simulink model "Simulacion_stepper_2024a"  (R2024a)
settings: Solver=ode4  StartTime=0.0  StopTime=Time_simulation  FixedStep=1/frecuency_simulation  RelTol=1e-3
InitFcn:
  | %%InitFcn();
StopFcn:
  | %%FinishFcn
model workspace (MAT data in the model file):
  Ts_stepper = 0.001
values from neighbouring files (symbols this model uses):
  B = motor_params.B_internal    [bode.m]    (also in current_observer.m = 0.0005; discretizacion.m = [ 1/L, 0; ekf_4_estados.m = params.B; obs_ctrl_back_emf_ext.m = [1/L 0)
  B0 = 3*wn_w - BJ_hat    [Barrido_B.m]    (also in Barrido_J.m; InitFcn.m = 449.962302294)
  B1 = 3*wn_w^2 - B0*BJ_hat    [Barrido_B.m]    (also in Barrido_J.m; InitFcn.m = 64448.3670019)
  B2 = -(J_var/P)*(wn_w^3)    [Barrido_B.m]    (also in Barrido_J.m; InitFcn.m = -0.364323750994)
  B_internal = 1e-4    (= 0.0001)    [InitFcn.m]
  B_var = B_internal* B_factors(k)    [Barrido_B.m]    (also in Barrido_J.m = B_real; InitFcn.m = 0.0001)
  frecuency_simulation = 10e3    (= 10000)    [InitFcn.m]
  I_nom = 1    [InitFcn.m]    (also in salient_motor.m)
  J = motor_params.J_internal    [bode.m]    (also in current_observer.m = 0.008; ekf_4_estados.m = params.J; obs_ctrl_back_emf_ext.m = 0.008; obs_y_contrl_back_emd.m = 0.008)
  J_internal = 4.7/1000000    (= 4.7e-06)    [InitFcn.m]
  J_var = J_real    [Barrido_B.m]    (also in Barrido_J.m = J_internal * J_factors(k); InitFcn.m = 4.7e-06)
  Ke = Kt    [InitFcn.m]    (also in current_observer.m = 0.0055; ekf_4_estados.m = params.Ke; observer.m = Pvec(3); salient_motor.m = 0.0066)
  Ki_d = wd_d*R    (= 3926.99081699)    [InitFcn.m]    (also in bode.m = PI_dq_params.Ki_d_salient)
  Ki_d_salient = wd_d^2*Ld    (= 21491.0635834)    [InitFcn.m]
  Ki_q = wd_q*R    (= 3926.99081699)    [InitFcn.m]    (also in bode.m = PI_dq_params.Ki_q_salient)
  Ki_q_salient = wd_q^2*Lq    (= 7846.33549887)    [InitFcn.m]
  Ki_w = (wn_w^2)*J_var/Kt    [Barrido_B.m]    (also in Barrido_J.m; InitFcn.m; bode.m = PI_MTPA_params.Ki_w)
  Kp_d = wd_d*L    (= 9.42477796077)    [InitFcn.m]    (also in bode.m = PI_dq_params.Kp_d_salient)
  Kp_d_salient = 2*shi_d*wd_d*Ld -R    (= 16.845833313)    [InitFcn.m]
  Kp_q = wd_q*L    (= 9.42477796077)    [InitFcn.m]    (also in bode.m = PI_dq_params.Kp_q_salient)
  Kp_q_salient = 2*shi_q*wd_q*Lq-R    (= 4.56311709936)    [InitFcn.m]
  Kp_w = (2*shi_w*wn_w*J_var)/Kt    [Barrido_B.m]    (also in Barrido_J.m; InitFcn.m; bode.m = PI_MTPA_params.Kp_w)
  Kt = Thold / (sqrt(2) * I_nom)    [InitFcn.m]    (also in current_observer.m = 0.275; ekf_4_estados.m = params.Kt; frecuencia_max.m = 0.33; observer.m = Pvec(4))
  L = 6/1000    (= 0.006)    [InitFcn.m]    (also in current_observer.m = place(A', C', 10*eig(A)).'; desfase.m = lags(k); discretizacion.m = 0.01; frecuencia_max.m)
  Ld = L0 + L2    [Copy_of_PMSM_salient.m]    (also in InitFcn.m = 0.00871; bode.m = motor_params.Ld; ekf_4_estados.m = params.Ld; salient_motor.m = 0.00871)
  Lq = L0 - L2    [Copy_of_PMSM_salient.m]    (also in InitFcn.m = 0.00318; bode.m = motor_params.Lq; ekf_4_estados.m = params.Lq; salient_motor.m = 0.00318)
  N_steps = 360/Step_angle    (= 200)    [InitFcn.m]
  P = N_teeths/2    (= 50)    [InitFcn.m]    (also in bode.m = motor_params.P; ekf_4_estados.m = P_pred; frecuencia_max.m; salient_motor.m)
  Phi = pi/2    (= 1.57079632679)    [InitFcn.m]    (also in ekf_4_estados.m = eye(4) + Ts_eff*A)
  Psi = Kt/P    [InitFcn.m]    (also in bode.m = motor_params.Ke; salient_motor.m = 0.0066)
  R = 2.5    [InitFcn.m]    (also in bode.m = motor_params.R; current_observer.m = 3.4; discretizacion.m = 3.4; ekf_4_estados.m = params.R)
  sample_time = 1/frecuency_simulation    (= 0.0001)    [InitFcn.m]
  Tdm = 18/1000    (= 0.018)    [InitFcn.m]    (also in salient_motor.m)
  Ts_current = 1/f_current    (= 0.0001)    [InitFcn.m]
  Ts_DO = Ts_Wm    (= 0.0001)    [InitFcn.m]
  Ts_ekf = 1/f_ekf    (= 0.0001)    [InitFcn.m]
  Ts_Wm = Ts_current    (= 0.0001)    [InitFcn.m]
  Vdc = 12    [InitFcn.m]    (also in frecuencia_max.m)
undefined symbols (not defined in the file or in its folder): DiscIntNeverNeededParam
libraries: fl_lib x27, nesl_utility x19, spsMosfetLib x16, simulink x8, eeTransforms x4, spsDCVoltageSourceLib x4, spsVoltageMeasurementLib x4, ee_lib x3, slexportprevious_tp74def212_4eb8_4616_a2bc_f4e795655e99 x1, spsTriangleGeneratorLib x1, spspowerguiLib x1
(part 2 of 4)

== system Simulacion_stepper_2024a/Meas 1 ==
  ERef : fl_lib/Electrical/Electrical Elements/Electrical Reference
  PS-Simulink Converter : nesl_utility/PS-Simulink Converter  PhysicalDomain=network_engine_domain  SubClassName=ps_output  LeftPortType=input  RightPortType=output  PseudoPeriodic=off  Frequencies=[]  VectorFormat=1-D array  Unit=V  AffineConversion=off
  Voltage Sensor : fl_lib/Electrical/Electrical Sensors/Voltage Sensor
  V : PMIOPort  Side=Left
  SL : Outport  VectorParamsAs1DForOutWhenUnconnected=off
  wires:
  PS-Simulink Converter/1 -> SL/1
  connections:
  V/RConn1 -- Voltage Sensor/LConn1
  ERef/LConn1 -- Voltage Sensor/RConn2
  Voltage Sensor/RConn1 -- PS-Simulink Converter/LConn1

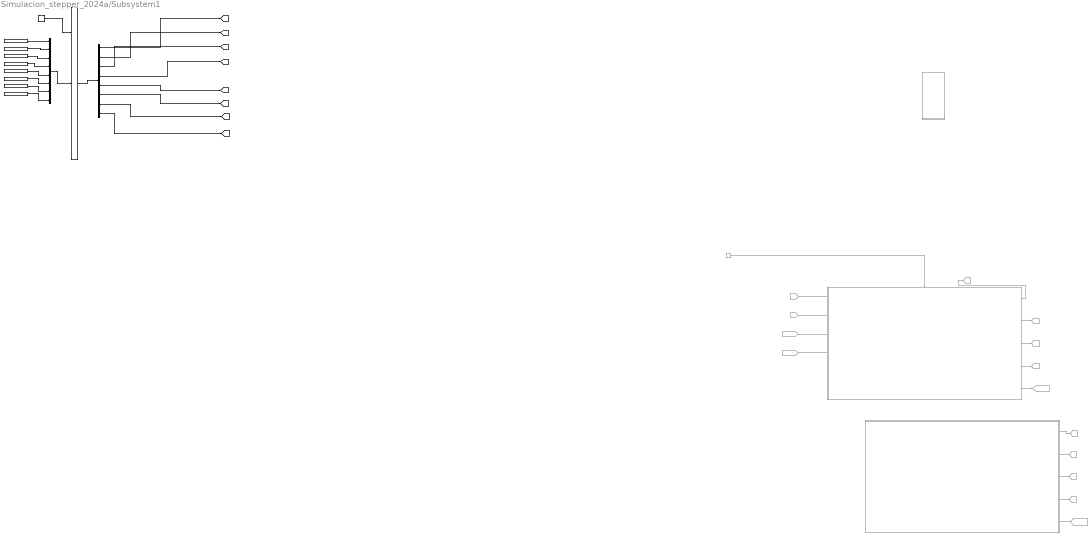
== system Simulacion_stepper_2024a/Subsystem1 ==
  note: A
  note: A
  note: A
  Constant1 : Constant
  Demux6 : Demux  Outputs=8
  From103 : From  Commented=on  GotoTag=Ib_M1
  From110 : From  Commented=on  GotoTag=Wm_ref  TagVisibility=global
  From112 : From  Commented=on  GotoTag=Wm_planta_M1  TagVisibility=global
  From98 : From  Commented=on  GotoTag=Ia_M1
  Function-Call Generator3 : FunctionCallGenerator  Commented=on  SampleTime=sample_time
  Goto14 : Goto  Commented=on  GotoTag=Vd_M2  TagVisibility=global
  Goto15 : Goto  Commented=on  GotoTag=Vq_M2  TagVisibility=global
  Goto16 : Goto  Commented=on  GotoTag=Iq_M2  TagVisibility=global
  Goto17 : Goto  Commented=on  GotoTag=Iq_ref_M2  TagVisibility=global
  Goto4 : Goto  Commented=on  GotoTag=Id_M2  TagVisibility=global
  Goto55 : Goto  Commented=on  GotoTag=Id_M1  TagVisibility=global
  Goto64 : Goto  Commented=on  GotoTag=Vd_M1  TagVisibility=global
  Goto65 : Goto  Commented=on  GotoTag=Vq_M1  TagVisibility=global
  Goto66 : Goto  Commented=on  GotoTag=Iq_M1  TagVisibility=global
  Goto68 : Goto  Commented=on  GotoTag=Iq_ref_M1  TagVisibility=global
  Multiport Switch : MultiPortSwitch  Inputs=2  SaturateOnIntegerOverflow=off  InputSameDT=off
  Mux1 : Mux  Inputs=8
  Repeating Sequence Stair : simulink/Sources/Repeating Sequence Stair  OutValues=[1 0 0 0]  tsamp=Ts_stepper  OutMin=[]  OutMax=[]  OutDataTypeStr=double  OutputDataTypeScalingMode=double  OutDataType=fixdt(0,8)  ConRadixGroup=Best Precision: Vector-wise  OutScaling=2^-12
  Repeating Sequence Stair1 : simulink/Sources/Repeating Sequence Stair  OutValues=[1 0 1 0]  tsamp=Ts_stepper  OutMin=[]  OutMax=[]  OutDataTypeStr=double  OutputDataTypeScalingMode=double  OutDataType=fixdt(0,8)  ConRadixGroup=Best Precision: Vector-wise  OutScaling=2^-12
  Repeating Sequence Stair10 : simulink/Sources/Repeating Sequence Stair  OutValues=[0 0 0 1]  tsamp=Ts_stepper  OutMin=[]  OutMax=[]  OutDataTypeStr=double  OutputDataTypeScalingMode=double  OutDataType=fixdt(0,8)  ConRadixGroup=Best Precision: Vector-wise  OutScaling=2^-12
  Repeating Sequence Stair11 : simulink/Sources/Repeating Sequence Stair  OutValues=[1 0 0 1]  tsamp=Ts_stepper  OutMin=[]  OutMax=[]  OutDataTypeStr=double  OutputDataTypeScalingMode=double  OutDataType=fixdt(0,8)  ConRadixGroup=Best Precision: Vector-wise  OutScaling=2^-12
  Repeating Sequence Stair2 : simulink/Sources/Repeating Sequence Stair  OutValues=[0 0 1 0]  tsamp=Ts_stepper  OutMin=[]  OutMax=[]  OutDataTypeStr=double  OutputDataTypeScalingMode=double  OutDataType=fixdt(0,8)  ConRadixGroup=Best Precision: Vector-wise  OutScaling=2^-12
  Repeating Sequence Stair3 : simulink/Sources/Repeating Sequence Stair  OutValues=[0 1 1 0]  tsamp=Ts_stepper  OutMin=[]  OutMax=[]  OutDataTypeStr=double  OutputDataTypeScalingMode=double  OutDataType=fixdt(0,8)  ConRadixGroup=Best Precision: Vector-wise  OutScaling=2^-12
  Repeating Sequence Stair8 : simulink/Sources/Repeating Sequence Stair  OutValues=[0 1 0 0]  tsamp=Ts_stepper  OutMin=[]  OutMax=[]  OutDataTypeStr=double  OutputDataTypeScalingMode=double  OutDataType=fixdt(0,8)  ConRadixGroup=Best Precision: Vector-wise  OutScaling=2^-12
  Repeating Sequence Stair9 : simulink/Sources/Repeating Sequence Stair  OutValues=[0 1 0 1]  tsamp=Ts_stepper  OutMin=[]  OutMax=[]  OutDataTypeStr=double  OutputDataTypeScalingMode=double  OutDataType=fixdt(0,8)  ConRadixGroup=Best Precision: Vector-wise  OutScaling=2^-12
  Subsystem : Subsystem  Commented=on
  Triggered Subsystem2 : Subsystem  Commented=on  TreatAsAtomicUnit=on
  Triggered Subsystem4 : Subsystem  Commented=on  TreatAsAtomicUnit=on
  wires:
  Triggered Subsystem2/4(Iq) -> Goto66/1
  Triggered Subsystem2/1(Vd) -> Goto64/1
  ? -> Triggered Subsystem4/6(Tl_Tdm)
  ? -> Triggered Subsystem2/5(Theta)
  ? -> Triggered Subsystem4/3(Wm_ref)
  Triggered Subsystem2/5(Iq_ref) -> Goto68/1
  From112/1 -> Triggered Subsystem2/4(Wm)
  Triggered Subsystem4/2(Vq) -> Goto15/1
  From98/1 -> Triggered Subsystem2/1(Ia)
  Triggered Subsystem2/2(Vq) -> Goto65/1
  ? -> Triggered Subsystem2/6(Tl_Tdm)
  From103/1 -> Triggered Subsystem2/2(Ib)
  Triggered Subsystem2/3(Id) -> Goto55/1
  From110/1 -> Triggered Subsystem2/3(Wm_ref)
  Triggered Subsystem4/3(Id) -> Goto4/1
  ? -> Triggered Subsystem4/Trigger
  Triggered Subsystem4/4(Iq) -> Goto16/1
  ? -> Triggered Subsystem4/4(Wm)
  Triggered Subsystem4/5(Iq_ref) -> Goto17/1
  ? -> Triggered Subsystem4/5(Theta)
  ? -> Triggered Subsystem4/1(Ia)
  Function-Call Generator3/1 -> Triggered Subsystem2/Trigger
  ? -> Triggered Subsystem4/2(Ib)
  Triggered Subsystem4/1(Vd) -> Goto14/1
  Demux6/2 -> [S2_M0]
  Demux6/1 -> [S1_M0]
  Repeating Sequence Stair10/1 -> Mux1/7
  Repeating Sequence Stair8/1 -> Mux1/5
  Repeating Sequence Stair9/1 -> Mux1/6
  Demux6/8 -> [S8_M0]
  Demux6/4 -> [S4_M0]
  Demux6/7 -> [S7_M0]
  Demux6/6 -> [S6_M0]
  Constant1/1 -> Multiport Switch/1
  Repeating Sequence Stair/1 -> Mux1/1
  Mux1/1 -> Multiport Switch/2
  Repeating Sequence Stair3/1 -> Mux1/4
  Repeating Sequence Stair11/1 -> Mux1/8
  Demux6/5 -> [S5_M0]
  Repeating Sequence Stair2/1 -> Mux1/3
  Repeating Sequence Stair1/1 -> Mux1/2
  Multiport Switch/1 -> Demux6/1
  Demux6/3 -> [S3_M0]

== system Simulacion_stepper_2024a/Triggered Subsystem ==
  Wm_cmd : Inport
  Trigger : TriggerPort  TriggerType=function-call  VariantControl=(inherit)
  Constant : Constant  Value=1/1000
  Constant1 : Constant  Value=0
  MATLAB Function : MATLAB Function  TreatAsAtomicUnit=on
  Wm_ref : Outport
  Alpha_ref : Outport  Port=2
  wires:
  MATLAB Function/1(Wm_ref) -> Wm_ref/1
  MATLAB Function/2(alpha_ref) -> Alpha_ref/1
  Wm_cmd/1 -> MATLAB Function/1(Wm_cmd)
  Constant/1 -> MATLAB Function/2(Ts)
  Constant1/1 -> MATLAB Function/3(slope)

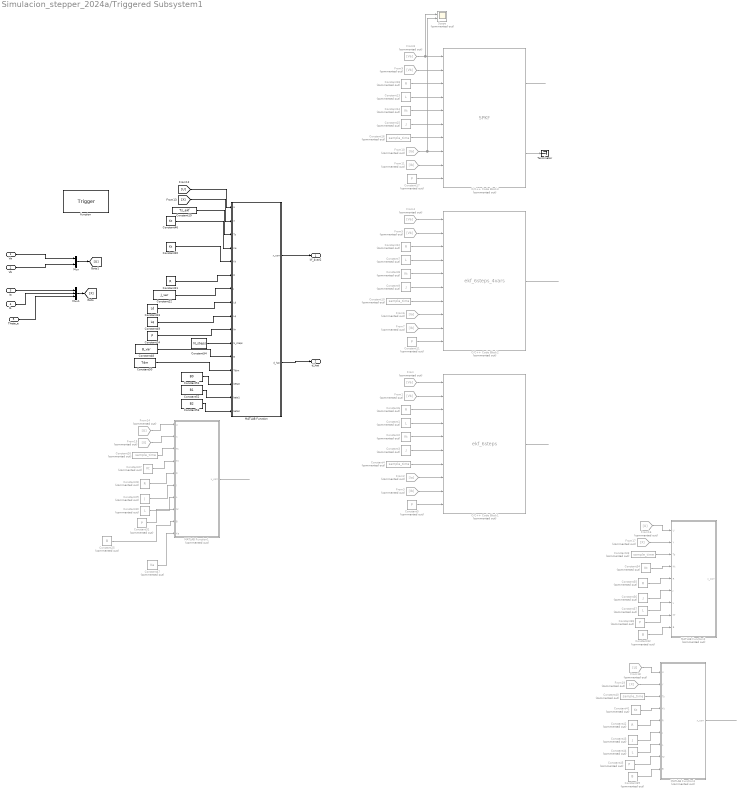
== system Simulacion_stepper_2024a/Triggered Subsystem1 ==
  Va : Inport
  Vb : Inport  Port=2
  Ia : Inport  Port=3
  Ib : Inport  Port=4
  Theta_e : Inport  Port=5
  function : TriggerPort  TriggerType=function-call  VariantControl=(inherit)  SampleTime=1/100
  C/C++ Code Block1 : S-Function  Commented=on  FunctionName=ekf_6steps  SFunctionModules=ekf_6steps_wrapper.c  SFunctionDeploymentMode=off  EnableBusSupport=off  mask(S-Function Builder){}
      mask help: Simulink:masks:SFunctionBuilder_MD
      mask init:
      | val = [[.9  0.75 0.75 1 1 .9 .9 1]',[1 1 0.75 0.75 .9 .9 1 .9]'];try , sys = get_param(gcb,'SfunBuilderFcnName');if isempty(sys), sys = get_param(gcb,'FunctionName'); end,catch, sys = get_param(gcb,'FunctionName'); end
      settings: CopyFcn=set_param(gcbh,'LinkStatus','none')  OpenFcn=sfunctionwizard(gcbh)
      mask Display:
      | plot(val(:,1),val(:,2))
      | disp(sys)
      | port_label('input',1,sprintf('%s', 'Va'),'interpreter','tex')
      | port_label('input',2,sprintf('%s', 'Vb'),'interpreter','tex')
      | port_label('input',3,sprintf('%s', 'R'),'interpreter','tex')
      | port_label('input',4,sprintf('%s', 'L'),'interpreter','tex')
      | port_label('input',5,sprintf('%s', 'Kt'),'interpreter','tex')
      | port_label('input',6,sprintf('%s', 'J'),'interpreter','tex')
      | port_label('input',7,sprintf('%s', 'Ts'),'interpreter','tex')
      | port_label('input',8,sprintf('%s', 'Ia\_medido'),'interpreter','tex')
      | port_label('input',9,sprintf('%s', 'Ib\_medido'),'interpreter','tex')
      | port_label('input',10,sprintf('%s', 'Nr'),'interpreter','tex')
      | port_label('output',1,sprintf('%s', 'x\_corr\_out'),'interpreter','tex')
  C/C++ Code Block2 : S-Function  Commented=on  FunctionName=ekf_6steps_4vars  SFunctionModules=ekf_6steps_4vars_wrapper.c  SFunctionDeploymentMode=off  EnableBusSupport=off  mask(S-Function Builder){}
      mask help: Simulink:masks:SFunctionBuilder_MD
      mask init: same as Simulacion_stepper_2024a/Triggered Subsystem1/C/C++ Code Block1
      settings: CopyFcn=set_param(gcbh,'LinkStatus','none')  OpenFcn=sfunctionwizard(gcbh)
      mask Display:
      | plot(val(:,1),val(:,2))
      | disp(sys)
      | port_label('input',1,sprintf('%s', 'Va'),'interpreter','tex')
      | port_label('input',2,sprintf('%s', 'Vb'),'interpreter','tex')
      | port_label('input',3,sprintf('%s', 'R'),'interpreter','tex')
      | port_label('input',4,sprintf('%s', 'L'),'interpreter','tex')
      | port_label('input',5,sprintf('%s', 'Kt'),'interpreter','tex')
      | port_label('input',6,sprintf('%s', 'J'),'interpreter','tex')
      | port_label('input',7,sprintf('%s', 'Ts'),'interpreter','tex')
      | port_label('input',8,sprintf('%s', 'Ia\_medido'),'interpreter','tex')
      | port_label('input',9,sprintf('%s', 'Ib\_medido'),'interpreter','tex')
      | port_label('input',10,sprintf('%s', 'Nr'),'interpreter','tex')
      | port_label('output',1,sprintf('%s', 'x\_corr\_out'),'interpreter','tex')
  C/C++ Code Block3 : S-Function  Commented=on  FunctionName=SPKF  SFunctionModules=SPKF_wrapper.c  SFunctionDeploymentMode=off  EnableBusSupport=off  mask(S-Function Builder){}
      mask help: Simulink:masks:SFunctionBuilder_MD
      mask init: same as Simulacion_stepper_2024a/Triggered Subsystem1/C/C++ Code Block1
      settings: CopyFcn=set_param(gcbh,'LinkStatus','none')  OpenFcn=sfunctionwizard(gcbh)
      mask Display:
      | plot(val(:,1),val(:,2))
      | disp(sys)
      | port_label('input',1,sprintf('%s', 'Va'),'interpreter','tex')
      | port_label('input',2,sprintf('%s', 'Vb'),'interpreter','tex')
      | port_label('input',3,sprintf('%s', 'R'),'interpreter','tex')
      | port_label('input',4,sprintf('%s', 'L'),'interpreter','tex')
      | port_label('input',5,sprintf('%s', 'Kt'),'interpreter','tex')
      | port_label('input',6,sprintf('%s', 'J'),'interpreter','tex')
      | port_label('input',7,sprintf('%s', 'Ts'),'interpreter','tex')
      | port_label('input',8,sprintf('%s', 'Ia\_medido'),'interpreter','tex')
      | port_label('input',9,sprintf('%s', 'Ib\_medido'),'interpreter','tex')
      | port_label('input',10,sprintf('%s', 'Nr'),'interpreter','tex')
      | port_label('output',1,sprintf('%s', 'x'),'interpreter','tex')
      | port_label('output',2,sprintf('%s', 'x\_aux'),'interpreter','tex')
  Constant{1,7,13,30,37,44} (6 alike) : Constant  Commented=on  Value=L  OutDataTypeStr=double
  Constant{4,10,16,26,33,40} (6 alike) : Constant  Commented=on  Value=sample_time  OutDataTypeStr=double
  Constant{5,11,17,31,38,45} (6 alike) : Constant  Commented=on  Value=P  OutDataTypeStr=double
  Constant{6,12,18,28,35,42} (6 alike) : Constant  Commented=on  Value=R  OutDataTypeStr=double
  Constant{2,8,14,27,34,41} (6 alike) : Constant  Commented=on  Value=Kt  OutDataTypeStr=double
  Constant{3,9,15,29,36,43} (6 alike) : Constant  Commented=on  Value=J  OutDataTypeStr=double
  Constant19 : Constant  Value=Ts_ekf  OutDataTypeStr=double
  Constant20 : Constant  Value=Kt  OutDataTypeStr=double
  Constant21 : Constant  Value=R  OutDataTypeStr=double
  Constant22 : Constant  Value=J_var  OutDataTypeStr=double
  Constant23 : Constant  Value=Ld  OutDataTypeStr=double
  Constant24 : Constant  Value=P  OutDataTypeStr=double
  Constant25 : Constant  Commented=on  Value=B
  Constant32 : Constant  Commented=on  Value=B
  Constant39 : Constant  Commented=on  Value=B
  Constant46 : Constant  Value=Kt  OutDataTypeStr=double
  Constant47 : Constant  Commented=on  Value=Ke  OutDataTypeStr=double
  Constant48 : Constant  Value=B_var  OutDataTypeStr=double
  Constant49 : Constant  Value=Lq  OutDataTypeStr=double
  Constant50 : Constant  Value=Tdm  OutDataTypeStr=double
  Constant51 : Constant  Value=B0  OutDataTypeStr=double
  Constant52 : Constant  Value=B1  OutDataTypeStr=double
  Constant53 : Constant  Value=B2  OutDataTypeStr=double
  Constant54 : Constant  Value=N_steps  OutDataTypeStr=double
  From : From  Commented=on  GotoTag=Va
  From1 : From  Commented=on  GotoTag=Vb
  From10 : From  Commented=on  GotoTag=Ia
  From11 : From  Commented=on  GotoTag=Ib
  From14 : From  Commented=on  GotoTag=U
  From15 : From  Commented=on  GotoTag=X
  From16 : From  Commented=on  GotoTag=U
  From17 : From  Commented=on  GotoTag=X
  From18 : From  Commented=on  GotoTag=U
  From19 : From  Commented=on  GotoTag=X
  From2 : From  Commented=on  GotoTag=Ia
  From3 : From  Commented=on  GotoTag=Ib
  From4 : From  Commented=on  GotoTag=Va
  From5 : From  Commented=on  GotoTag=Vb
  From6 : From  Commented=on  GotoTag=Ia
  From7 : From  Commented=on  GotoTag=Ib
  From8 : From  Commented=on  GotoTag=Va
  From9 : From  Commented=on  GotoTag=Vb
  MATLAB Function : MATLAB Function  TreatAsAtomicUnit=on
  MATLAB Function1 : MATLAB Function  Commented=on  TreatAsAtomicUnit=on
  MATLAB Function2 : MATLAB Function  Commented=on  TreatAsAtomicUnit=on
  MATLAB Function3 : MATLAB Function  Commented=on  TreatAsAtomicUnit=on
  Mux : Mux  Inputs=2
  Mux1 : Mux  Inputs=3
  Scope : Scope  Commented=on  NumInputPorts=2
  Terminator : Terminator
  kf_4var2 : Outport  PortDimensions=[4 1]
  d_hat : Outport  Port=2
  wires:
  Constant4/1 -> C/C++ Code Block1/7
  Constant5/1 -> C/C++ Code Block1/10
  C/C++ Code Block1/1 -> ?
  Constant6/1 -> C/C++ Code Block1/3
  Constant1/1 -> C/C++ Code Block1/4
  Constant2/1 -> C/C++ Code Block1/5
  Constant3/1 -> C/C++ Code Block1/6
  C/C++ Code Block2/1 -> ?
  C/C++ Code Block3/1 -> ?
  Vb/1 -> Mux/2
  Va/1 -> Mux/1
  Ib/1 -> Mux1/2
  Ia/1 -> Mux1/1
  From/1 -> C/C++ Code Block1/1
  From1/1 -> C/C++ Code Block1/2
  From2/1 -> C/C++ Code Block1/8
  From3/1 -> C/C++ Code Block1/9
  From4/1 -> C/C++ Code Block2/1
  From7/1 -> C/C++ Code Block2/9
  Constant8/1 -> C/C++ Code Block2/5
  Constant12/1 -> C/C++ Code Block2/3
  From5/1 -> C/C++ Code Block2/2
  Constant11/1 -> C/C++ Code Block2/10
  From6/1 -> C/C++ Code Block2/8
  Constant9/1 -> C/C++ Code Block2/6
  Constant7/1 -> C/C++ Code Block2/4
  Constant10/1 -> C/C++ Code Block2/7
  From8/1 -> Scope/1, C/C++ Code Block3/1
  From11/1 -> C/C++ Code Block3/9
  Constant14/1 -> C/C++ Code Block3/5
  Constant18/1 -> C/C++ Code Block3/3
  From9/1 -> C/C++ Code Block3/2
  Constant17/1 -> C/C++ Code Block3/10
  From10/1 -> Scope/2, C/C++ Code Block3/8
  Constant15/1 -> C/C++ Code Block3/6
  Constant13/1 -> C/C++ Code Block3/4
  Constant16/1 -> C/C++ Code Block3/7
  C/C++ Code Block3/2 -> Terminator/1
  Mux1/1 -> [X]
  Mux/1 -> [U]
  From16/1 -> MATLAB Function2/1(U)
  From17/1 -> MATLAB Function2/2(Y)
  Constant33/1 -> MATLAB Function2/3(Ts)
  Constant32/1 -> MATLAB Function2/9(B)
  Constant37/1 -> MATLAB Function2/7(L)
  Constant35/1 -> MATLAB Function2/5(R)
  Constant36/1 -> MATLAB Function2/6(J)
  Constant34/1 -> MATLAB Function2/4(Kt)
  Constant38/1 -> MATLAB Function2/8(Nr)
  MATLAB Function3/1(x_corr) -> ?
  Constant45/1 -> MATLAB Function3/8(Nr)
  Constant41/1 -> MATLAB Function3/4(Kt)
  From19/1 -> MATLAB Function3/2(Y)
  Constant43/1 -> MATLAB Function3/6(J)
  Constant40/1 -> MATLAB Function3/3(Ts)
  Constant39/1 -> MATLAB Function3/9(B)
  Constant42/1 -> MATLAB Function3/5(R)
  From18/1 -> MATLAB Function3/1(U)
  Constant44/1 -> MATLAB Function3/7(L)
  From15/1 -> MATLAB Function1/2(X)
  Constant27/1 -> MATLAB Function1/4(Kt)
  Constant31/1 -> MATLAB Function1/8(Nr)
  Constant29/1 -> MATLAB Function1/6(J)
  Constant25/1 -> MATLAB Function1/9(B)
  Constant26/1 -> MATLAB Function1/3(Ts)
  Constant30/1 -> MATLAB Function1/7(L)
  Constant28/1 -> MATLAB Function1/5(R)
  From14/1 -> MATLAB Function1/1(U)
  Constant47/1 -> MATLAB Function1/10(Ke)
  MATLAB Function1/1(x_corr) -> ?
  [U] -> MATLAB Function/1(U)
  [X] -> MATLAB Function/2(X)
  Constant19/1 -> MATLAB Function/3(Ts)
  Constant46/1 -> MATLAB Function/4(Ke)
  Constant20/1 -> MATLAB Function/5(Kt)
  Constant21/1 -> MATLAB Function/6(R)
  Constant22/1 -> MATLAB Function/7(J)
  Constant23/1 -> MATLAB Function/8(Ld)
  Constant49/1 -> MATLAB Function/9(Lq)
  Constant24/1 -> MATLAB Function/10(Nr)
  Constant48/1 -> MATLAB Function/12(B)
  Constant50/1 -> MATLAB Function/13(Tdtm)
  MATLAB Function/1(x_corr) -> kf_4var2/1
  Theta_e/1 -> Mux1/3
  Constant51/1 -> MATLAB Function/14(beta0)
  Constant52/1 -> MATLAB Function/15(beta1)
  Constant53/1 -> MATLAB Function/16(beta2)
  MATLAB Function/2(d_hat) -> d_hat/1
  Constant54/1 -> MATLAB Function/11(N_steps)

== system Simulacion_stepper_2024a/Triggered Subsystem10 ==
  Wm_ref : Inport
  Wm : Inport  Port=2
  Tl_Tdm : Inport  Port=3
  theta_e : Inport  Port=4
  function : TriggerPort  TriggerType=function-call  VariantControl=(inherit)  SampleTime=1/100
  C/C++ Code Block : S-Function  Commented=on  FunctionName=PI_dq  SFunctionModules=PI_dq_wrapper.c  SFunctionDeploymentMode=off  EnableBusSupport=off  mask(S-Function Builder){}
      mask help: Simulink:masks:SFunctionBuilder_MD
      mask init: same as Simulacion_stepper_2024a/Triggered Subsystem1/C/C++ Code Block1
      settings: CopyFcn=set_param(gcbh,'LinkStatus','none')  OpenFcn=sfunctionwizard(gcbh)
      mask Display:
      | plot(val(:,1),val(:,2))
      | disp(sys)
      | port_label('input',1,sprintf('%s', 'Ia'),'interpreter','tex')
      | port_label('input',2,sprintf('%s', 'Ib'),'interpreter','tex')
      | port_label('input',3,sprintf('%s', 'Wm\_ref'),'interpreter','tex')
      | port_label('input',4,sprintf('%s', 'Wm\_ext'),'interpreter','tex')
      | port_label('input',5,sprintf('%s', 'Kp\_current'),'interpreter','tex')
      | port_label('input',6,sprintf('%s', 'Ki\_current'),'interpreter','tex')
      | port_label('input',7,sprintf('%s', 'Kd\_current'),'interpreter','tex')
      | port_label('input',8,sprintf('%s', 'sample\_time\_ext'),'interpreter','tex')
      | port_label('input',9,sprintf('%s', 'Vdc\_ext'),'interpreter','tex')
      | port_label('input',10,sprintf('%s', 'R\_ext'),'interpreter','tex')
      | port_label('input',11,sprintf('%s', 'Ld\_ext'),'interpreter','tex')
      | port_label('input',12,sprintf('%s', 'Lq\_ext'),'interpreter','tex')
      | port_label('input',13,sprintf('%s', 'Ke\_ext'),'interpreter','tex')
      | port_label('input',14,sprintf('%s', 'Theta\_ext'),'interpreter','tex')
      | port_label('input',15,sprintf('%s', 'Kp\_wm'),'interpreter','tex')
      | port_label('input',16,sprintf('%s', 'Ki\_wm'),'interpreter','tex')
      | port_label('input',17,sprintf('%s', 'Tl\_Tdm'),'interpreter','tex')
      | port_label('input',18,sprintf('%s', 'B'),'interpreter','tex')
      | port_label('input',19,sprintf('%s', 'Kt\_ext'),'interpreter','tex')
      | port_label('output',1,sprintf('%s', 'Ud'),'interpreter','tex')
      | port_label('output',2,sprintf('%s', 'Uq'),'interpreter','tex')
      | port_label('output',3,sprintf('%s', 'Id'),'interpreter','tex')
      | port_label('output',4,sprintf('%s', 'Iq'),'interpreter','tex')
      | port_label('output',5,sprintf('%s', 'Iq\_ref\_aux'),'interpreter','tex')
  Constant : Constant  Value=B_var  OutDataTypeStr=double
  Constant1 : Constant  Value=Kp_w  OutDataTypeStr=double
  Constant11 : Constant  Value=Ki_w  OutDataTypeStr=double
  Constant12 : Constant  Value=Kt  OutDataTypeStr=double
  Constant2 : Constant  Value=I_nom  OutDataTypeStr=double
  Constant3 : Constant  Value=Ts_Wm  OutDataTypeStr=double
  Constant4 : Constant  Value=Tdm  OutDataTypeStr=double
  MATLAB Function : MATLAB Function  TreatAsAtomicUnit=on
  Iq_ref : Outport
  Wm_filt_out : Outport  Port=2
  wires:
  MATLAB Function/1(Iq_ref) -> Iq_ref/1
  Wm_ref/1 -> MATLAB Function/1(Wm_ref)
  Wm/1 -> MATLAB Function/2(Wm)
  Constant12/1 -> MATLAB Function/8(Kt)
  Constant/1 -> MATLAB Function/7(B)
  Tl_Tdm/1 -> MATLAB Function/6(Tl_tdm)
  Constant1/1 -> MATLAB Function/4(Kp_w)
  Constant11/1 -> MATLAB Function/5(Ki_w)
  Constant3/1 -> MATLAB Function/3(Ts)
  Constant2/1 -> MATLAB Function/11(Imax)
  theta_e/1 -> MATLAB Function/9(theta_e)
  Constant4/1 -> MATLAB Function/10(Tdm)
  MATLAB Function/2(Wm_filt_out) -> Wm_filt_out/1

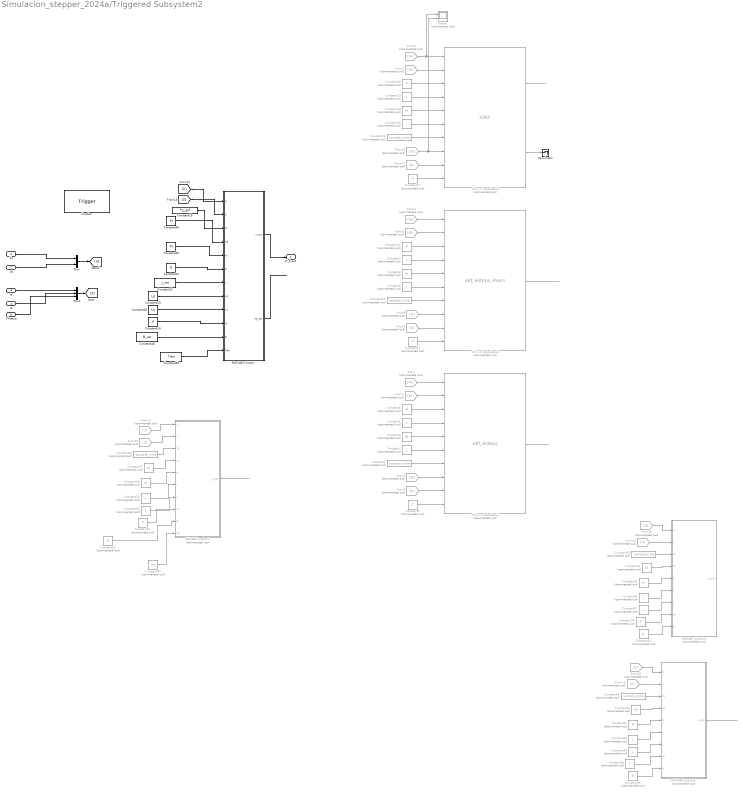
== system Simulacion_stepper_2024a/Triggered Subsystem2 ==
  Va : Inport
  Vb : Inport  Port=2
  Ia : Inport  Port=3
  Ib : Inport  Port=4
  Theta_e : Inport  Port=5
  function : TriggerPort  TriggerType=function-call  VariantControl=(inherit)  SampleTime=1/100
  C/C++ Code Block1 : S-Function  Commented=on  FunctionName=ekf_6steps  SFunctionModules=ekf_6steps_wrapper.c  SFunctionDeploymentMode=off  EnableBusSupport=off  mask(S-Function Builder){}
      mask help: Simulink:masks:SFunctionBuilder_MD
      mask init: same as Simulacion_stepper_2024a/Triggered Subsystem1/C/C++ Code Block1
      settings: CopyFcn=set_param(gcbh,'LinkStatus','none')  OpenFcn=sfunctionwizard(gcbh)
      mask Display:
      | plot(val(:,1),val(:,2))
      | disp(sys)
      | port_label('input',1,sprintf('%s', 'Va'),'interpreter','tex')
      | port_label('input',2,sprintf('%s', 'Vb'),'interpreter','tex')
      | port_label('input',3,sprintf('%s', 'R'),'interpreter','tex')
      | port_label('input',4,sprintf('%s', 'L'),'interpreter','tex')
      | port_label('input',5,sprintf('%s', 'Kt'),'interpreter','tex')
      | port_label('input',6,sprintf('%s', 'J'),'interpreter','tex')
      | port_label('input',7,sprintf('%s', 'Ts'),'interpreter','tex')
      | port_label('input',8,sprintf('%s', 'Ia\_medido'),'interpreter','tex')
      | port_label('input',9,sprintf('%s', 'Ib\_medido'),'interpreter','tex')
      | port_label('input',10,sprintf('%s', 'Nr'),'interpreter','tex')
      | port_label('output',1,sprintf('%s', 'x\_corr\_out'),'interpreter','tex')
  C/C++ Code Block2 : S-Function  Commented=on  FunctionName=ekf_6steps_4vars  SFunctionModules=ekf_6steps_4vars_wrapper.c  SFunctionDeploymentMode=off  EnableBusSupport=off  mask(S-Function Builder){}
      mask help: Simulink:masks:SFunctionBuilder_MD
      mask init: same as Simulacion_stepper_2024a/Triggered Subsystem1/C/C++ Code Block1
      settings: CopyFcn=set_param(gcbh,'LinkStatus','none')  OpenFcn=sfunctionwizard(gcbh)
      mask Display:
      | plot(val(:,1),val(:,2))
      | disp(sys)
      | port_label('input',1,sprintf('%s', 'Va'),'interpreter','tex')
      | port_label('input',2,sprintf('%s', 'Vb'),'interpreter','tex')
      | port_label('input',3,sprintf('%s', 'R'),'interpreter','tex')
      | port_label('input',4,sprintf('%s', 'L'),'interpreter','tex')
      | port_label('input',5,sprintf('%s', 'Kt'),'interpreter','tex')
      | port_label('input',6,sprintf('%s', 'J'),'interpreter','tex')
      | port_label('input',7,sprintf('%s', 'Ts'),'interpreter','tex')
      | port_label('input',8,sprintf('%s', 'Ia\_medido'),'interpreter','tex')
      | port_label('input',9,sprintf('%s', 'Ib\_medido'),'interpreter','tex')
      | port_label('input',10,sprintf('%s', 'Nr'),'interpreter','tex')
      | port_label('output',1,sprintf('%s', 'x\_corr\_out'),'interpreter','tex')
  C/C++ Code Block3 : S-Function  Commented=on  FunctionName=SPKF  SFunctionModules=SPKF_wrapper.c  SFunctionDeploymentMode=off  EnableBusSupport=off  mask(S-Function Builder){}
      mask help: Simulink:masks:SFunctionBuilder_MD
      mask init: same as Simulacion_stepper_2024a/Triggered Subsystem1/C/C++ Code Block1
      settings: CopyFcn=set_param(gcbh,'LinkStatus','none')  OpenFcn=sfunctionwizard(gcbh)
      mask Display:
      | plot(val(:,1),val(:,2))
      | disp(sys)
      | port_label('input',1,sprintf('%s', 'Va'),'interpreter','tex')
      | port_label('input',2,sprintf('%s', 'Vb'),'interpreter','tex')
      | port_label('input',3,sprintf('%s', 'R'),'interpreter','tex')
      | port_label('input',4,sprintf('%s', 'L'),'interpreter','tex')
      | port_label('input',5,sprintf('%s', 'Kt'),'interpreter','tex')
      | port_label('input',6,sprintf('%s', 'J'),'interpreter','tex')
      | port_label('input',7,sprintf('%s', 'Ts'),'interpreter','tex')
      | port_label('input',8,sprintf('%s', 'Ia\_medido'),'interpreter','tex')
      | port_label('input',9,sprintf('%s', 'Ib\_medido'),'interpreter','tex')
      | port_label('input',10,sprintf('%s', 'Nr'),'interpreter','tex')
      | port_label('output',1,sprintf('%s', 'x'),'interpreter','tex')
      | port_label('output',2,sprintf('%s', 'x\_aux'),'interpreter','tex')
  Constant{1,7,13,30,37,44} (6 alike) : Constant  Commented=on  Value=L  OutDataTypeStr=double
  Constant{4,10,16,26,33,40} (6 alike) : Constant  Commented=on  Value=sample_time  OutDataTypeStr=double
  Constant{5,11,17,31,38,45} (6 alike) : Constant  Commented=on  Value=P  OutDataTypeStr=double
  Constant{6,12,18,28,35,42} (6 alike) : Constant  Commented=on  Value=R  OutDataTypeStr=double
  Constant{2,8,14,27,34,41} (6 alike) : Constant  Commented=on  Value=Kt  OutDataTypeStr=double
  Constant{3,9,15,29,36,43} (6 alike) : Constant  Commented=on  Value=J  OutDataTypeStr=double
  Constant19 : Constant  Value=Ts_ekf  OutDataTypeStr=double
  Constant20 : Constant  Value=Kt  OutDataTypeStr=double
  Constant21 : Constant  Value=R  OutDataTypeStr=double
  Constant22 : Constant  Value=J_var  OutDataTypeStr=double
  Constant23 : Constant  Value=Ld  OutDataTypeStr=double
  Constant24 : Constant  Value=P  OutDataTypeStr=double
  Constant25 : Constant  Commented=on  Value=B
  Constant32 : Constant  Commented=on  Value=B
  Constant39 : Constant  Commented=on  Value=B
  Constant46 : Constant  Value=Kt  OutDataTypeStr=double
  Constant47 : Constant  Commented=on  Value=Ke  OutDataTypeStr=double
  Constant48 : Constant  Value=B_var  OutDataTypeStr=double
  Constant49 : Constant  Value=Lq  OutDataTypeStr=double
  Constant50 : Constant  Value=Tdm  OutDataTypeStr=double
  From : From  Commented=on  GotoTag=Va
  From1 : From  Commented=on  GotoTag=Vb
  From10 : From  Commented=on  GotoTag=Ia
  From11 : From  Commented=on  GotoTag=Ib
  From14 : From  Commented=on  GotoTag=U
  From15 : From  Commented=on  GotoTag=X
  From16 : From  Commented=on  GotoTag=U
  From17 : From  Commented=on  GotoTag=X
  From18 : From  Commented=on  GotoTag=U
  From19 : From  Commented=on  GotoTag=X
  From2 : From  Commented=on  GotoTag=Ia
  From3 : From  Commented=on  GotoTag=Ib
  From4 : From  Commented=on  GotoTag=Va
  From5 : From  Commented=on  GotoTag=Vb
  From6 : From  Commented=on  GotoTag=Ia
  From7 : From  Commented=on  GotoTag=Ib
  From8 : From  Commented=on  GotoTag=Va
  From9 : From  Commented=on  GotoTag=Vb
  MATLAB Function : MATLAB Function  TreatAsAtomicUnit=on
  MATLAB Function1 : MATLAB Function  Commented=on  TreatAsAtomicUnit=on
  MATLAB Function2 : MATLAB Function  Commented=on  TreatAsAtomicUnit=on
  MATLAB Function3 : MATLAB Function  Commented=on  TreatAsAtomicUnit=on
  Mux : Mux  Inputs=2
  Mux1 : Mux  Inputs=3
  Scope : Scope  Commented=on  NumInputPorts=2
  Terminator : Terminator
  kf_4var2 : Outport
  wires:
  Constant4/1 -> C/C++ Code Block1/7
  Constant5/1 -> C/C++ Code Block1/10
  C/C++ Code Block1/1 -> ?
  Constant6/1 -> C/C++ Code Block1/3
  Constant1/1 -> C/C++ Code Block1/4
  Constant2/1 -> C/C++ Code Block1/5
  Constant3/1 -> C/C++ Code Block1/6
  C/C++ Code Block2/1 -> ?
  C/C++ Code Block3/1 -> ?
  Vb/1 -> Mux/2
  Va/1 -> Mux/1
  Ib/1 -> Mux1/2
  Ia/1 -> Mux1/1
  From/1 -> C/C++ Code Block1/1
  From1/1 -> C/C++ Code Block1/2
  From2/1 -> C/C++ Code Block1/8
  From3/1 -> C/C++ Code Block1/9
  From4/1 -> C/C++ Code Block2/1
  From7/1 -> C/C++ Code Block2/9
  Constant8/1 -> C/C++ Code Block2/5
  Constant12/1 -> C/C++ Code Block2/3
  From5/1 -> C/C++ Code Block2/2
  Constant11/1 -> C/C++ Code Block2/10
  From6/1 -> C/C++ Code Block2/8
  Constant9/1 -> C/C++ Code Block2/6
  Constant7/1 -> C/C++ Code Block2/4
  Constant10/1 -> C/C++ Code Block2/7
  From8/1 -> Scope/1, C/C++ Code Block3/1
  From11/1 -> C/C++ Code Block3/9
  Constant14/1 -> C/C++ Code Block3/5
  Constant18/1 -> C/C++ Code Block3/3
  From9/1 -> C/C++ Code Block3/2
  Constant17/1 -> C/C++ Code Block3/10
  From10/1 -> Scope/2, C/C++ Code Block3/8
  Constant15/1 -> C/C++ Code Block3/6
  Constant13/1 -> C/C++ Code Block3/4
  Constant16/1 -> C/C++ Code Block3/7
  C/C++ Code Block3/2 -> Terminator/1
  Mux1/1 -> [X]
  Mux/1 -> [U]
  [U] -> MATLAB Function/1(U)
  [X] -> MATLAB Function/2(X)
  Constant19/1 -> MATLAB Function/3(Ts)
  Constant20/1 -> MATLAB Function/5(Kt)
  Constant21/1 -> MATLAB Function/6(R)
  Constant22/1 -> MATLAB Function/7(J)
  Constant23/1 -> MATLAB Function/8(Ld)
  Constant24/1 -> MATLAB Function/10(Nr)
  From16/1 -> MATLAB Function2/1(U)
  From17/1 -> MATLAB Function2/2(Y)
  Constant33/1 -> MATLAB Function2/3(Ts)
  Constant32/1 -> MATLAB Function2/9(B)
  Constant37/1 -> MATLAB Function2/7(L)
  Constant35/1 -> MATLAB Function2/5(R)
  Constant36/1 -> MATLAB Function2/6(J)
  Constant34/1 -> MATLAB Function2/4(Kt)
  Constant38/1 -> MATLAB Function2/8(Nr)
  MATLAB Function3/1(x_corr) -> ?
  Constant45/1 -> MATLAB Function3/8(Nr)
  Constant41/1 -> MATLAB Function3/4(Kt)
  From19/1 -> MATLAB Function3/2(Y)
  Constant43/1 -> MATLAB Function3/6(J)
  Constant40/1 -> MATLAB Function3/3(Ts)
  Constant39/1 -> MATLAB Function3/9(B)
  Constant42/1 -> MATLAB Function3/5(R)
  From18/1 -> MATLAB Function3/1(U)
  Constant44/1 -> MATLAB Function3/7(L)
  Constant46/1 -> MATLAB Function/4(Ke)
  From15/1 -> MATLAB Function1/2(X)
  Constant27/1 -> MATLAB Function1/4(Kt)
  Constant31/1 -> MATLAB Function1/8(Nr)
  Constant29/1 -> MATLAB Function1/6(J)
  Constant25/1 -> MATLAB Function1/9(B)
  Constant26/1 -> MATLAB Function1/3(Ts)
  Constant30/1 -> MATLAB Function1/7(L)
  Constant28/1 -> MATLAB Function1/5(R)
  From14/1 -> MATLAB Function1/1(U)
  Constant47/1 -> MATLAB Function1/10(Ke)
  MATLAB Function1/1(x_corr) -> ?
  MATLAB Function/1(x_corr) -> kf_4var2/1
  Constant48/1 -> MATLAB Function/11(B)
  MATLAB Function/2(Te_est) -> ?
  Theta_e/1 -> Mux1/3
  Constant49/1 -> MATLAB Function/9(Lq)
  Constant50/1 -> MATLAB Function/12(Tdm)

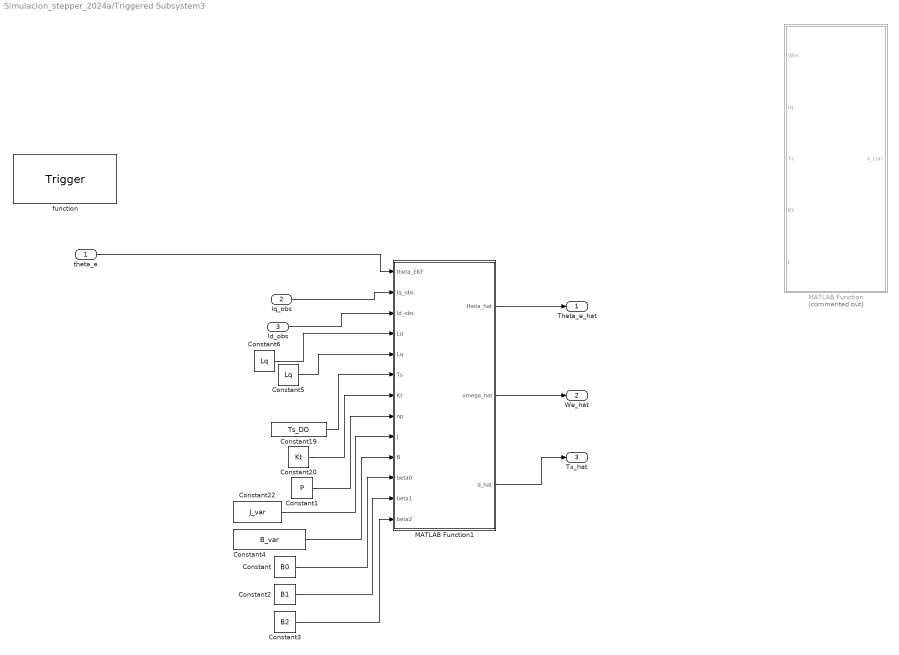
== system Simulacion_stepper_2024a/Triggered Subsystem3 ==
  theta_e : Inport
  Iq_obs : Inport  Port=2
  Id_obs : Inport  Port=3
  function : TriggerPort  TriggerType=function-call  VariantControl=(inherit)  SampleTime=1/100
  Constant : Constant  Value=B0
  Constant1 : Constant  Value=P  OutDataTypeStr=double
  Constant19 : Constant  Value=Ts_DO  OutDataTypeStr=double
  Constant2 : Constant  Value=B1
  Constant20 : Constant  Value=Kt  OutDataTypeStr=double
  Constant22 : Constant  Value=J_var  OutDataTypeStr=double
  Constant3 : Constant  Value=B2
  Constant4 : Constant  Value=B_var  OutDataTypeStr=double
  Constant5 : Constant  Value=Lq
  Constant6 : Constant  Value=Lq
  MATLAB Function : MATLAB Function  Commented=on  TreatAsAtomicUnit=on
  MATLAB Function1 : MATLAB Function  TreatAsAtomicUnit=on
  Theta_e_hat : Outport
  We_hat : Outport  Port=2
  Tx_hat : Outport  Port=3  PortDimensions=1
  wires:
  theta_e/1 -> MATLAB Function1/1(theta_EKF)
  MATLAB Function1/1(theta_hat) -> Theta_e_hat/1
  MATLAB Function1/2(omega_hat) -> We_hat/1
  Constant19/1 -> MATLAB Function1/6(Ts)
  Constant20/1 -> MATLAB Function1/7(Kt)
  Constant1/1 -> MATLAB Function1/8(np)
  Constant22/1 -> MATLAB Function1/9(J)
  Constant4/1 -> MATLAB Function1/10(B)
  Constant/1 -> MATLAB Function1/11(beta0)
  Constant2/1 -> MATLAB Function1/12(beta1)
  Constant3/1 -> MATLAB Function1/13(beta2)
  MATLAB Function1/3(d_hat) -> Tx_hat/1
  Iq_obs/1 -> MATLAB Function1/2(Iq_obs)
  Id_obs/1 -> MATLAB Function1/3(Id_obs)
  Constant5/1 -> MATLAB Function1/5(Lq)
  Constant6/1 -> MATLAB Function1/4(Ld)

== system Simulacion_stepper_2024a/Triggered Subsystem4 ==
  theta_e : Inport
  Iq_obs : Inport  Port=2
  function : TriggerPort  TriggerType=function-call  VariantControl=(inherit)  SampleTime=1/100
  Constant : Constant  Value=B0
  Constant1 : Constant  Value=P  OutDataTypeStr=double
  Constant19 : Constant  Value=Ts_DO  OutDataTypeStr=double
  Constant2 : Constant  Value=B1
  Constant20 : Constant  Value=Kt  OutDataTypeStr=double
  Constant22 : Constant  Value=J_var  OutDataTypeStr=double
  Constant3 : Constant  Value=B2
  Constant4 : Constant  Value=B_var  OutDataTypeStr=double
  MATLAB Function : MATLAB Function  Commented=on  TreatAsAtomicUnit=on
  MATLAB Function1 : MATLAB Function  TreatAsAtomicUnit=on
  Theta_e_hat : Outport
  We_hat : Outport  Port=2
  Tx_hat : Outport  Port=3
  wires:
  theta_e/1 -> MATLAB Function1/1(theta_EKF)
  MATLAB Function1/1(theta_hat) -> Theta_e_hat/1
  MATLAB Function1/2(omega_hat) -> We_hat/1
  Constant19/1 -> MATLAB Function1/3(Ts)
  Constant20/1 -> MATLAB Function1/4(Kt)
  Constant1/1 -> MATLAB Function1/5(np)
  Constant22/1 -> MATLAB Function1/6(J)
  Constant4/1 -> MATLAB Function1/7(B)
  Constant/1 -> MATLAB Function1/8(beta0)
  Constant2/1 -> MATLAB Function1/9(beta1)
  Constant3/1 -> MATLAB Function1/10(beta2)
  MATLAB Function1/3(d_hat) -> Tx_hat/1
  Iq_obs/1 -> MATLAB Function1/2(Iq_obs)

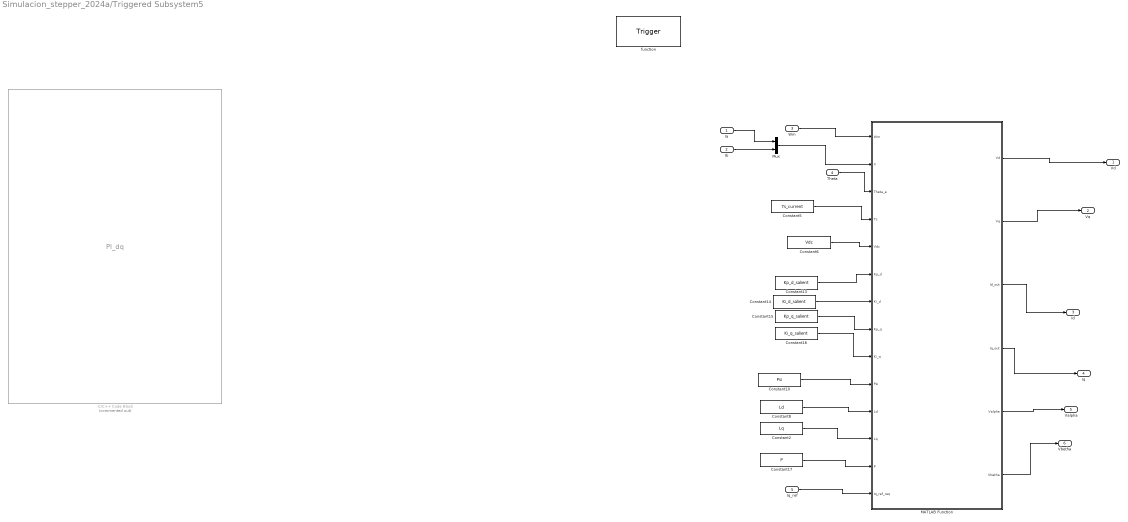
== system Simulacion_stepper_2024a/Triggered Subsystem5 ==
  Ia : Inport  PortDimensions=1
  Ib : Inport  Port=2  PortDimensions=1
  Wm : Inport  Port=3
  Theta : Inport  Port=4
  Iq_ref : Inport  Port=5
  function : TriggerPort  TriggerType=function-call  VariantControl=(inherit)  SampleTime=1/100
  C/C++ Code Block : S-Function  Commented=on  FunctionName=PI_dq  SFunctionModules=PI_dq_wrapper.c  SFunctionDeploymentMode=off  EnableBusSupport=off  mask(S-Function Builder){}
      mask help: Simulink:masks:SFunctionBuilder_MD
      mask init: same as Simulacion_stepper_2024a/Triggered Subsystem1/C/C++ Code Block1
      settings: CopyFcn=set_param(gcbh,'LinkStatus','none')  OpenFcn=sfunctionwizard(gcbh)
      mask Display:
      | plot(val(:,1),val(:,2))
      | disp(sys)
      | port_label('input',1,sprintf('%s', 'Ia'),'interpreter','tex')
      | port_label('input',2,sprintf('%s', 'Ib'),'interpreter','tex')
      | port_label('input',3,sprintf('%s', 'Wm\_ref'),'interpreter','tex')
      | port_label('input',4,sprintf('%s', 'Wm\_ext'),'interpreter','tex')
      | port_label('input',5,sprintf('%s', 'Kp\_current'),'interpreter','tex')
      | port_label('input',6,sprintf('%s', 'Ki\_current'),'interpreter','tex')
      | port_label('input',7,sprintf('%s', 'Kd\_current'),'interpreter','tex')
      | port_label('input',8,sprintf('%s', 'sample\_time\_ext'),'interpreter','tex')
      | port_label('input',9,sprintf('%s', 'Vdc\_ext'),'interpreter','tex')
      | port_label('input',10,sprintf('%s', 'R\_ext'),'interpreter','tex')
      | port_label('input',11,sprintf('%s', 'Ld\_ext'),'interpreter','tex')
      | port_label('input',12,sprintf('%s', 'Lq\_ext'),'interpreter','tex')
      | port_label('input',13,sprintf('%s', 'Ke\_ext'),'interpreter','tex')
      | port_label('input',14,sprintf('%s', 'Theta\_ext'),'interpreter','tex')
      | port_label('input',15,sprintf('%s', 'Kp\_wm'),'interpreter','tex')
      | port_label('input',16,sprintf('%s', 'Ki\_wm'),'interpreter','tex')
      | port_label('input',17,sprintf('%s', 'Tl\_Tdm'),'interpreter','tex')
      | port_label('input',18,sprintf('%s', 'B'),'interpreter','tex')
      | port_label('input',19,sprintf('%s', 'Kt\_ext'),'interpreter','tex')
      | port_label('output',1,sprintf('%s', 'Ud'),'interpreter','tex')
      | port_label('output',2,sprintf('%s', 'Uq'),'interpreter','tex')
      | port_label('output',3,sprintf('%s', 'Id'),'interpreter','tex')
      | port_label('output',4,sprintf('%s', 'Iq'),'interpreter','tex')
      | port_label('output',5,sprintf('%s', 'Iq\_ref\_aux'),'interpreter','tex')
  Constant10 : Constant  Value=Psi  OutDataTypeStr=double
  Constant13 : Constant  Value=Kp_d_salient  OutDataTypeStr=double
  Constant14 : Constant  Value=Ki_d_salient  OutDataTypeStr=double
  Constant15 : Constant  Value=Kp_q_salient  OutDataTypeStr=double
  Constant16 : Constant  Value=Ki_q_salient  OutDataTypeStr=double
  Constant17 : Constant  Value=P  OutDataTypeStr=double
  Constant2 : Constant  Value=Lq  OutDataTypeStr=double
  Constant5 : Constant  Value=Ts_current  OutDataTypeStr=double
  Constant6 : Constant  Value=Vdc  OutDataTypeStr=double
  Constant8 : Constant  Value=Ld  OutDataTypeStr=double
  MATLAB Function : MATLAB Function  TreatAsAtomicUnit=on
  Mux : Mux  Inputs=2
  Vd : Outport  PortDimensions=1
  Vq : Outport  Port=2  PortDimensions=1
  Id : Outport  Port=3
  Iq : Outport  Port=4
  Valpha : Outport  Port=5
  Vbetha : Outport  Port=6
  wires:
  MATLAB Function/1(Vd) -> Vd/1
  Wm/1 -> MATLAB Function/1(Wm)
  Ia/1 -> Mux/1
  Ib/1 -> Mux/2
  Mux/1 -> MATLAB Function/2(X)
  Theta/1 -> MATLAB Function/3(Theta_e)
  Constant5/1 -> MATLAB Function/4(Ts)
  Constant6/1 -> MATLAB Function/5(Vdc)
  Constant13/1 -> MATLAB Function/6(Kp_d)
  Constant14/1 -> MATLAB Function/7(Ki_d)
  Constant15/1 -> MATLAB Function/8(Kp_q)
  Constant16/1 -> MATLAB Function/9(Ki_q)
  Constant10/1 -> MATLAB Function/10(Psi)
  Constant8/1 -> MATLAB Function/11(Ld)
  Constant17/1 -> MATLAB Function/13(P)
  Constant2/1 -> MATLAB Function/12(Lq)
  MATLAB Function/2(Vq) -> Vq/1
  MATLAB Function/3(Id_out) -> Id/1
  MATLAB Function/4(Iq_out) -> Iq/1
  Iq_ref/1 -> MATLAB Function/14(Iq_ref_req)
  MATLAB Function/5(Valpha) -> Valpha/1
  MATLAB Function/6(Vbetha) -> Vbetha/1

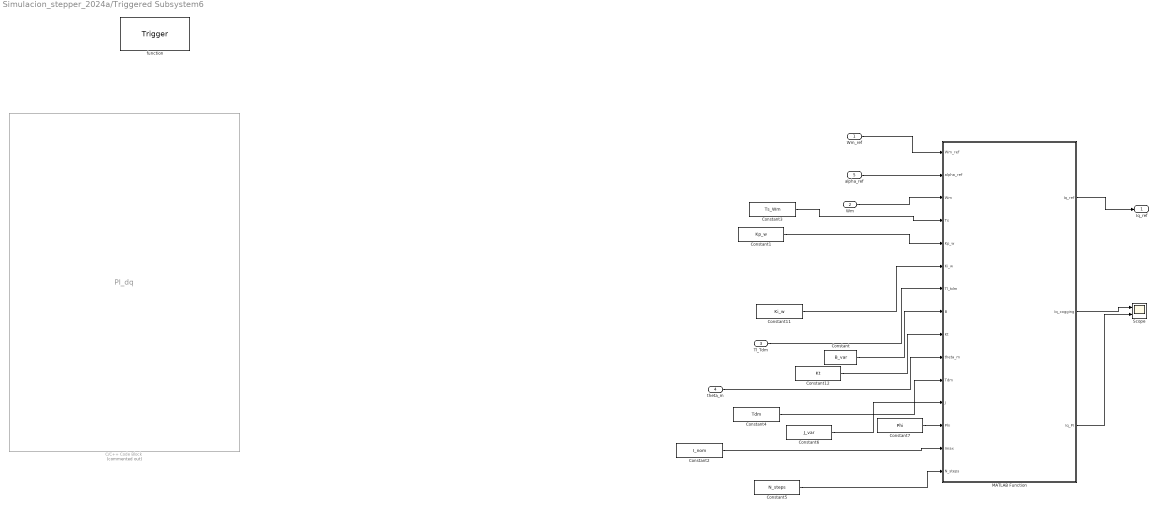
== system Simulacion_stepper_2024a/Triggered Subsystem6 ==
  Wm_ref : Inport
  Wm : Inport  Port=2
  Tl_Tdm : Inport  Port=3  PortDimensions=[1 1]
  theta_m : Inport  Port=4
  alpha_ref : Inport  Port=5
  function : TriggerPort  TriggerType=function-call  VariantControl=(inherit)  SampleTime=1/100
  C/C++ Code Block : S-Function  Commented=on  FunctionName=PI_dq  SFunctionModules=PI_dq_wrapper.c  SFunctionDeploymentMode=off  EnableBusSupport=off  mask(S-Function Builder){}
      mask help: Simulink:masks:SFunctionBuilder_MD
      mask init: same as Simulacion_stepper_2024a/Triggered Subsystem1/C/C++ Code Block1
      settings: CopyFcn=set_param(gcbh,'LinkStatus','none')  OpenFcn=sfunctionwizard(gcbh)
      mask Display:
      | plot(val(:,1),val(:,2))
      | disp(sys)
      | port_label('input',1,sprintf('%s', 'Ia'),'interpreter','tex')
      | port_label('input',2,sprintf('%s', 'Ib'),'interpreter','tex')
      | port_label('input',3,sprintf('%s', 'Wm\_ref'),'interpreter','tex')
      | port_label('input',4,sprintf('%s', 'Wm\_ext'),'interpreter','tex')
      | port_label('input',5,sprintf('%s', 'Kp\_current'),'interpreter','tex')
      | port_label('input',6,sprintf('%s', 'Ki\_current'),'interpreter','tex')
      | port_label('input',7,sprintf('%s', 'Kd\_current'),'interpreter','tex')
      | port_label('input',8,sprintf('%s', 'sample\_time\_ext'),'interpreter','tex')
      | port_label('input',9,sprintf('%s', 'Vdc\_ext'),'interpreter','tex')
      | port_label('input',10,sprintf('%s', 'R\_ext'),'interpreter','tex')
      | port_label('input',11,sprintf('%s', 'Ld\_ext'),'interpreter','tex')
      | port_label('input',12,sprintf('%s', 'Lq\_ext'),'interpreter','tex')
      | port_label('input',13,sprintf('%s', 'Ke\_ext'),'interpreter','tex')
      | port_label('input',14,sprintf('%s', 'Theta\_ext'),'interpreter','tex')
      | port_label('input',15,sprintf('%s', 'Kp\_wm'),'interpreter','tex')
      | port_label('input',16,sprintf('%s', 'Ki\_wm'),'interpreter','tex')
      | port_label('input',17,sprintf('%s', 'Tl\_Tdm'),'interpreter','tex')
      | port_label('input',18,sprintf('%s', 'B'),'interpreter','tex')
      | port_label('input',19,sprintf('%s', 'Kt\_ext'),'interpreter','tex')
      | port_label('output',1,sprintf('%s', 'Ud'),'interpreter','tex')
      | port_label('output',2,sprintf('%s', 'Uq'),'interpreter','tex')
      | port_label('output',3,sprintf('%s', 'Id'),'interpreter','tex')
      | port_label('output',4,sprintf('%s', 'Iq'),'interpreter','tex')
      | port_label('output',5,sprintf('%s', 'Iq\_ref\_aux'),'interpreter','tex')
  Constant : Constant  Value=B_var  OutDataTypeStr=double
  Constant1 : Constant  Value=Kp_w  OutDataTypeStr=double
  Constant11 : Constant  Value=Ki_w  OutDataTypeStr=double
  Constant12 : Constant  Value=Kt  OutDataTypeStr=double
  Constant2 : Constant  Value=I_nom  OutDataTypeStr=double
  Constant3 : Constant  Value=Ts_Wm  OutDataTypeStr=double
  Constant4 : Constant  Value=Tdm  OutDataTypeStr=double
  Constant5 : Constant  Value=N_steps  OutDataTypeStr=double
  Constant6 : Constant  Value=J_var  OutDataTypeStr=double
  Constant7 : Constant  Value=Phi  OutDataTypeStr=double
  MATLAB Function : MATLAB Function  TreatAsAtomicUnit=on
  Scope : Scope  NumInputPorts=2
  Iq_ref : Outport
  wires:
  MATLAB Function/1(Iq_ref) -> Iq_ref/1
  Wm_ref/1 -> MATLAB Function/1(Wm_ref)
  Wm/1 -> MATLAB Function/3(Wm)
  Constant12/1 -> MATLAB Function/9(Kt)
  Constant/1 -> MATLAB Function/8(B)
  Tl_Tdm/1 -> MATLAB Function/7(Tl_tdm)
  Constant1/1 -> MATLAB Function/5(Kp_w)
  Constant11/1 -> MATLAB Function/6(Ki_w)
  Constant3/1 -> MATLAB Function/4(Ts)
  Constant2/1 -> MATLAB Function/14(Imax)
  theta_m/1 -> MATLAB Function/10(theta_m)
  Constant4/1 -> MATLAB Function/11(Tdm)
  Constant5/1 -> MATLAB Function/15(N_steps)
  alpha_ref/1 -> MATLAB Function/2(alpha_ref)
  Constant6/1 -> MATLAB Function/12(J)
  MATLAB Function/2(Iq_cogging) -> Scope/1
  MATLAB Function/3(Iq_PI) -> Scope/2
  Constant7/1 -> MATLAB Function/13(Phi)

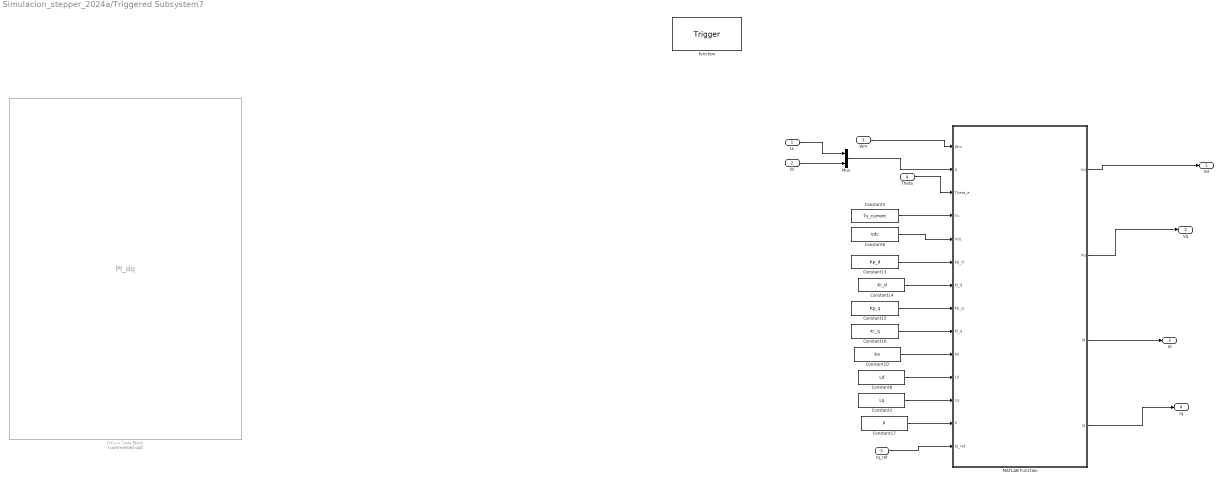
== system Simulacion_stepper_2024a/Triggered Subsystem7 ==
  Ia : Inport
  Ib : Inport  Port=2
  Wm : Inport  Port=3
  Theta : Inport  Port=4
  Iq_ref : Inport  Port=5
  function : TriggerPort  TriggerType=function-call  VariantControl=(inherit)  SampleTime=1/100
  C/C++ Code Block : S-Function  Commented=on  FunctionName=PI_dq  SFunctionModules=PI_dq_wrapper.c  SFunctionDeploymentMode=off  EnableBusSupport=off  mask(S-Function Builder){}
      mask help: Simulink:masks:SFunctionBuilder_MD
      mask init: same as Simulacion_stepper_2024a/Triggered Subsystem1/C/C++ Code Block1
      settings: CopyFcn=set_param(gcbh,'LinkStatus','none')  OpenFcn=sfunctionwizard(gcbh)
      mask Display:
      | plot(val(:,1),val(:,2))
      | disp(sys)
      | port_label('input',1,sprintf('%s', 'Ia'),'interpreter','tex')
      | port_label('input',2,sprintf('%s', 'Ib'),'interpreter','tex')
      | port_label('input',3,sprintf('%s', 'Wm\_ref'),'interpreter','tex')
      | port_label('input',4,sprintf('%s', 'Wm\_ext'),'interpreter','tex')
      | port_label('input',5,sprintf('%s', 'Kp\_current'),'interpreter','tex')
      | port_label('input',6,sprintf('%s', 'Ki\_current'),'interpreter','tex')
      | port_label('input',7,sprintf('%s', 'Kd\_current'),'interpreter','tex')
      | port_label('input',8,sprintf('%s', 'sample\_time\_ext'),'interpreter','tex')
      | port_label('input',9,sprintf('%s', 'Vdc\_ext'),'interpreter','tex')
      | port_label('input',10,sprintf('%s', 'R\_ext'),'interpreter','tex')
      | port_label('input',11,sprintf('%s', 'Ld\_ext'),'interpreter','tex')
      | port_label('input',12,sprintf('%s', 'Lq\_ext'),'interpreter','tex')
      | port_label('input',13,sprintf('%s', 'Ke\_ext'),'interpreter','tex')
      | port_label('input',14,sprintf('%s', 'Theta\_ext'),'interpreter','tex')
      | port_label('input',15,sprintf('%s', 'Kp\_wm'),'interpreter','tex')
      | port_label('input',16,sprintf('%s', 'Ki\_wm'),'interpreter','tex')
      | port_label('input',17,sprintf('%s', 'Tl\_Tdm'),'interpreter','tex')
      | port_label('input',18,sprintf('%s', 'B'),'interpreter','tex')
      | port_label('input',19,sprintf('%s', 'Kt\_ext'),'interpreter','tex')
      | port_label('output',1,sprintf('%s', 'Ud'),'interpreter','tex')
      | port_label('output',2,sprintf('%s', 'Uq'),'interpreter','tex')
      | port_label('output',3,sprintf('%s', 'Id'),'interpreter','tex')
      | port_label('output',4,sprintf('%s', 'Iq'),'interpreter','tex')
      | port_label('output',5,sprintf('%s', 'Iq\_ref\_aux'),'interpreter','tex')
  Constant10 : Constant  Value=Ke  OutDataTypeStr=double
  Constant13 : Constant  Value=Kp_d  OutDataTypeStr=double
  Constant14 : Constant  Value=Ki_d  OutDataTypeStr=double
  Constant15 : Constant  Value=Kp_q  OutDataTypeStr=double
  Constant16 : Constant  Value=Ki_q  OutDataTypeStr=double
  Constant17 : Constant  Value=P  OutDataTypeStr=double
  Constant2 : Constant  Value=Lq  OutDataTypeStr=double
  Constant5 : Constant  Value=Ts_current  OutDataTypeStr=double
  Constant6 : Constant  Value=Vdc  OutDataTypeStr=double
  Constant8 : Constant  Value=Ld  OutDataTypeStr=double
  MATLAB Function : MATLAB Function  TreatAsAtomicUnit=on
  Mux : Mux  Inputs=2
  Vd : Outport
  Vq : Outport  Port=2
  Id : Outport  Port=3
  Iq : Outport  Port=4
  wires:
  MATLAB Function/1(Vd) -> Vd/1
  Wm/1 -> MATLAB Function/1(Wm)
  Ia/1 -> Mux/1
  Ib/1 -> Mux/2
  Mux/1 -> MATLAB Function/2(X)
  Theta/1 -> MATLAB Function/3(Theta_e)
  Constant5/1 -> MATLAB Function/4(Ts)
  Constant6/1 -> MATLAB Function/5(Vdc)
  Constant13/1 -> MATLAB Function/6(Kp_d)
  Constant14/1 -> MATLAB Function/7(Ki_d)
  Constant15/1 -> MATLAB Function/8(Kp_q)
  Constant16/1 -> MATLAB Function/9(Ki_q)
  Constant10/1 -> MATLAB Function/10(Ke)
  Constant8/1 -> MATLAB Function/11(Ld)
  Constant17/1 -> MATLAB Function/13(P)
  Constant2/1 -> MATLAB Function/12(Lq)
  MATLAB Function/2(Vq) -> Vq/1
  MATLAB Function/3(Id) -> Id/1
  MATLAB Function/4(Iq) -> Iq/1
  Iq_ref/1 -> MATLAB Function/14(Iq_ref)
